simulink model "finalsimple_VER"  (R2023b)
settings: Solver=VariableStepAuto  StartTime=0.0  StopTime=5  FixedStep=4  MaxStep=0.01  RelTol=1e-3
undefined symbols (not defined in the file or in its folder): Ion, Lithium
libraries: simulink x40, nesl_utility x10, spsSeriesRLCBranchLib x8, fl_lib x6, spsMosfetLib x6, dspsrcs4 x5, spsControlledCurrentSourceLib x5, ee_lib x4, spsCurrentMeasurementLib x4, spsVoltageMeasurementLib x4, spsBatteryLib x3, spsGroundLib x2
(part 2 of 2)

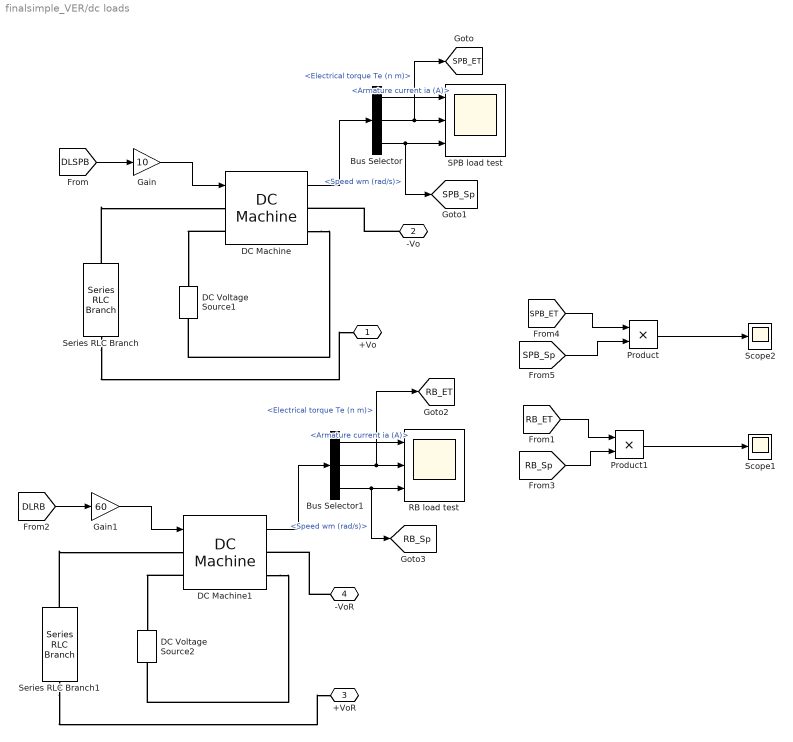
== system finalsimple_VER/dc loads ==
  Bus Selector : BusSelector  OutputSignals=Armature current ia (A),Electrical torque Te (n m),Speed wm (rad/s)
  Bus Selector1 : BusSelector  OutputSignals=Armature current ia (A),Electrical torque Te (n m),Speed wm (rad/s)
  DC Machine : spsDCMachineLib/DC Machine  PresetModel=No  MechanicalLoad=Speed w  FieldType=Wound  ShowDetailedParameters=on  MeasurementBus=off  RLa=[0.2828 0.004453]  RLf=[69.77 9.413]  Laf=0.5899  MachineConstant=Torque constant (N.m/A)  Ke=1.8  Kt=1.8  J=1.019  Bm=0.02516  Tf=26.46  w0=1  Ifinit=-8.59968467822847  TsPowergui=0  TsBlock=1
  DC Machine1 : spsDCMachineLib/DC Machine  PresetModel=No  MechanicalLoad=Speed w  FieldType=Wound  ShowDetailedParameters=on  MeasurementBus=off  RLa=[0.2828 0.004453]  RLf=[69.77 9.413]  Laf=0.5899  MachineConstant=Torque constant (N.m/A)  Ke=1.8  Kt=1.8  J=1.019  Bm=0.02516  Tf=26.46  w0=1  Ifinit=-4.29984233911423  TsPowergui=0  TsBlock=1
  DC Voltage Source1 : spsDCVoltageSourceLib/DC Voltage Source  Amplitude=600  Measurements=None
  DC Voltage Source2 : spsDCVoltageSourceLib/DC Voltage Source  Amplitude=300  Measurements=None
  Gain : Gain  Gain=10
  Gain1 : Gain  Gain=60
  Product : Product
  Product1 : Product
  RB load test : Scope  NumInputPorts=3
  SPB load test : Scope  NumInputPorts=3
  Scope1 : Scope
  Scope2 : Scope
  Series RLC Branch : spsSeriesRLCBranchLib/Series RLC Branch  LConnTagsString=__new0  RConnTagsString=__new0  BranchType=R  Resistance=1e3  Inductance=1e-3  SetiL0=off  InitialCurrent=0  Capacitance=1e-6  Setx0=off  InitialVoltage=0  Measurements=None
  Series RLC Branch1 : spsSeriesRLCBranchLib/Series RLC Branch  LConnTagsString=__new0  RConnTagsString=__new0  BranchType=R  Resistance=1e3  Inductance=1e-3  SetiL0=off  InitialCurrent=0  Capacitance=1e-6  Setx0=off  InitialVoltage=0  Measurements=None
  +Vo : PMIOPort  Side=Right
  -Vo : PMIOPort  Port=2  Side=Right
  +VoR : PMIOPort  Port=3  Side=Right
  -VoR : PMIOPort  Port=4  Side=Right
  tag scope: RB_ET=global, RB_Sp=global, SPB_ET=global, SPB_Sp=global
  wires:
  Bus Selector/3 -> SPB load test/3, [SPB_Sp]  "<Speed wm (rad/s)>"
  Bus Selector/2 -> [SPB_ET], SPB load test/2  "<Electrical torque Te (n m)>"
  DC Machine/1 -> Bus Selector/1
  Bus Selector/1 -> SPB load test/1  "<Armature current ia (A)>"
  [DLSPB] -> Gain/1
  [DLRB] -> Gain1/1
  Bus Selector1/1 -> RB load test/1  "<Armature current ia (A)>"
  DC Machine1/1 -> Bus Selector1/1
  Bus Selector1/2 -> [RB_ET], RB load test/2  "<Electrical torque Te (n m)>"
  Bus Selector1/3 -> [RB_Sp], RB load test/3  "<Speed wm (rad/s)>"
  Gain1/1 -> DC Machine1/1
  Gain/1 -> DC Machine/1
  [SPB_ET] -> Product/1
  [SPB_Sp] -> Product/2
  Product/1 -> Scope2/1
  Product1/1 -> Scope1/1
  [RB_ET] -> Product1/1
  [RB_Sp] -> Product1/2
  connections:
  -Vo/RConn1 -- DC Machine/RConn1
  DC Machine/RConn2 -- DC Voltage Source1/RConn1
  DC Machine/LConn2 -- DC Voltage Source1/LConn1
  Series RLC Branch/LConn1 -- DC Machine/LConn1
  Series RLC Branch1/LConn1 -- DC Machine1/LConn1
  DC Machine1/LConn2 -- DC Voltage Source2/LConn1
  DC Machine1/RConn2 -- DC Voltage Source2/RConn1
  -VoR/RConn1 -- DC Machine1/RConn1
  Series RLC Branch/RConn1 -- +Vo/RConn1
  Series RLC Branch1/RConn1 -- +VoR/RConn1

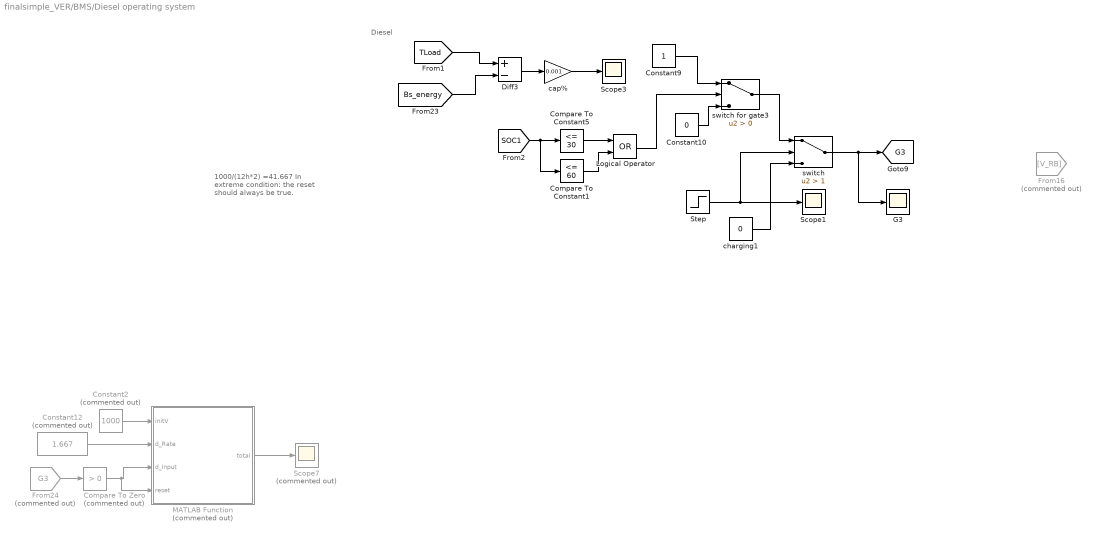
== system finalsimple_VER/BMS/Diesel operating system ==
  note: Diesel
  note: 1000/(12h*2)
      | =41.667
      |
      | In extreme condition:
      | the reset should
      | always be true.
  Compare To Constant1 : simulink/Logic and Bit Operations/Compare To Constant  relop=<=  const=60  OutDataTypeStr=boolean
  Compare To Constant5 : simulink/Logic and Bit Operations/Compare To Constant  relop=<=  const=30  OutDataTypeStr=boolean
  Compare To Zero : simulink/Logic and Bit Operations/Compare To Zero  Commented=on  relop=>  OutDataTypeStr=boolean
  Constant10 : Constant  Value=0
  Constant12 : Constant  Commented=on  Value=1.667
  Constant2 : Constant  Commented=on  Value=1000
  Constant9 : Constant
  Diff3 : Sum  Inputs=+-
  From16 : From  Commented=on  GotoTag=V_RB  TagVisibility=global
  From24 : From  Commented=on  GotoTag=G3  TagVisibility=global
  G3 : Scope
  Logical Operator : Logic  Operator=OR  AllPortsSameDT=off  OutDataTypeStr=boolean
  MATLAB Function : MATLAB Function  Commented=on  TreatAsAtomicUnit=on
  Scope1 : Scope
  Scope3 : Scope
  Scope7 : Scope  Commented=on
  Step : Step  Time=2400  After=2  SampleTime=1
  cap% : Gain  Gain=0.001
  charging1 : Constant  Value=0
  "switch " : Switch  Criteria=u2 > Threshold  Threshold=1  SaturateOnIntegerOverflow=off  InputSameDT=off
  switch for gate3 : Switch  Criteria=u2 > Threshold  SaturateOnIntegerOverflow=off  InputSameDT=off
  tag scope: G3=global
  wires:
  Constant9/1 -> switch for gate3/1
  Constant10/1 -> switch for gate3/3
  Constant12/1 -> MATLAB Function/2(d_Rate)
  MATLAB Function/1(total) -> Scope7/1
  Compare To Zero/1 -> MATLAB Function/4(reset), MATLAB Function/3(d_Input)
  From24/1 -> Compare To Zero/1
  Diff3/1 -> cap%/1
  Constant2/1 -> MATLAB Function/1(initV)
  [TLoad] -> Diff3/1
  Step/1 -> "switch "/2, Scope1/1
  charging1/1 -> "switch "/3
  "switch "/1 -> [G3], G3/1
  switch for gate3/1 -> "switch "/1
  [Bs_energy] -> Diff3/2
  [SOC1] -> Compare To Constant1/1, Compare To Constant5/1
  cap%/1 -> Scope3/1
  Compare To Constant1/1 -> Logical Operator/2
  Compare To Constant5/1 -> Logical Operator/1
  Logical Operator/1 -> switch for gate3/2

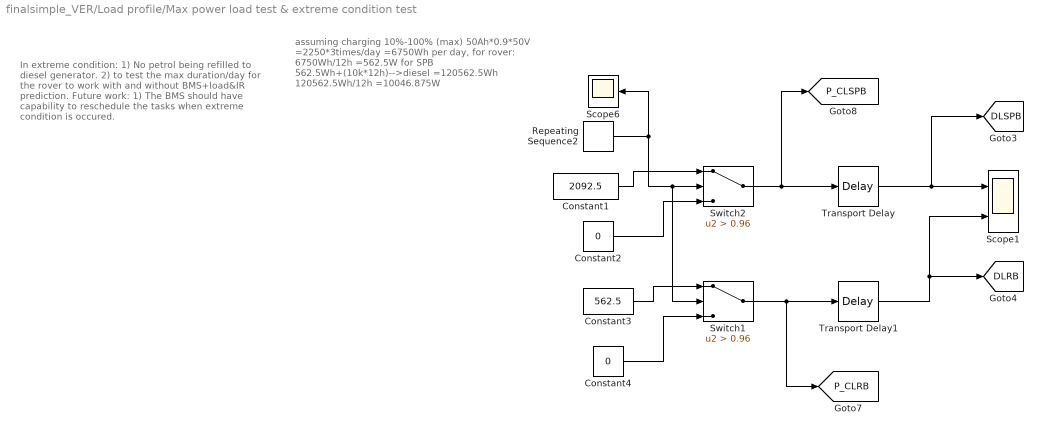
== system finalsimple_VER/Load profile/Max power load test & extreme condition test ==
  note: assuming charging 10%-100% (max)
      | 50Ah*0.9*50V
      | =2250*3times/day
      | =6750Wh per day,
      | for rover:
      | 6750Wh/12h
      | =562.5W
      |
      | for SPB
      | 562.5Wh+(10k*12h)-->diesel
      | =120562.5Wh
      |
      | 120562.5Wh/12h
      | =10046.875W
  note: In extreme condition:
      | 1) No petrol being refilled
      | to diesel generator.
      | 2) to test the max duration/day for
      | the rover to work with
      | and without BMS+load&IR prediction.
      |
      | Future work:
      | 1) The BMS should have capability
      | to reschedule the tasks when
      | extreme condition is occured.
  Constant1 : Constant  Value=2092.5
  Constant2 : Constant  Value=0
  Constant3 : Constant  Value=562.5
  Constant4 : Constant  Value=0
  Repeating Sequence2 : simulink/Sources/Repeating Sequence  rep_seq_t=[0 300 300.1 900.99 901 1200]  rep_seq_y=[0.9 0.9 1.01 1.01 0.9 0.9]
  Scope1 : Scope  NumInputPorts=2
  Scope6 : Scope
  Switch1 : Switch  Criteria=u2 > Threshold  Threshold=0.96  RndMeth=Ceiling  ZeroCross=off  SaturateOnIntegerOverflow=off
  Switch2 : Switch  Criteria=u2 > Threshold  Threshold=0.96  RndMeth=Ceiling  ZeroCross=off  SaturateOnIntegerOverflow=off
  Transport Delay : TransportDelay  DelayTime=2400
  Transport Delay1 : TransportDelay  DelayTime=2400
  tag scope: DLRB=global, DLSPB=global, P_CLRB=global, P_CLSPB=global
  wires:
  Switch1/1 -> [P_CLRB], Transport Delay1/1
  Switch2/1 -> [P_CLSPB], Transport Delay/1
  Repeating Sequence2/1 -> Scope6/1, Switch1/2, Switch2/2
  Constant2/1 -> Switch2/3
  Constant1/1 -> Switch2/1
  Constant3/1 -> Switch1/1
  Constant4/1 -> Switch1/3
  Transport Delay/1 -> [DLSPB], Scope1/1
  Transport Delay1/1 -> Scope1/2, [DLRB]

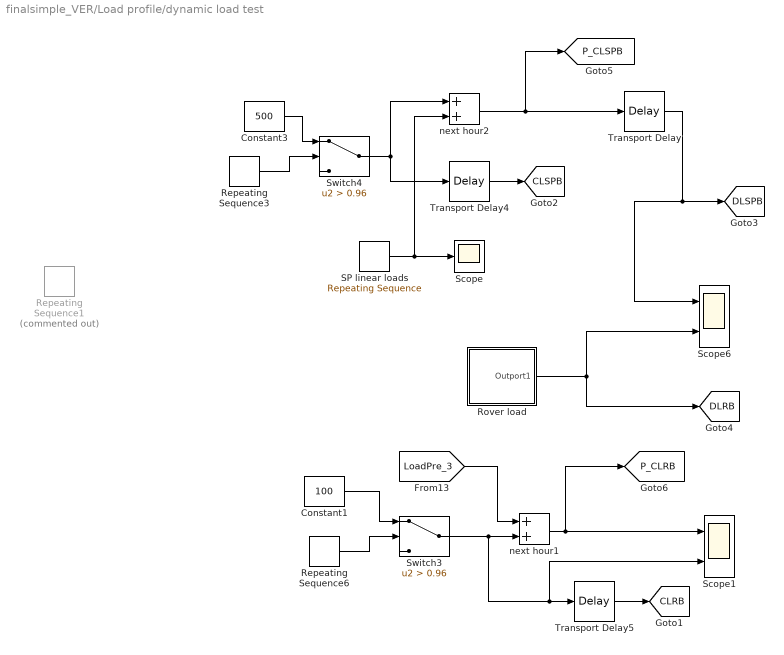
== system finalsimple_VER/Load profile/dynamic load test ==
  Constant1 : Constant  Value=100
  Constant3 : Constant  Value=500
  Repeating Sequence1 : simulink/Sources/Repeating Sequence  Commented=on  rep_seq_t=[0 400 500 600 700 800 900 1000 1200]  rep_seq_y=[0 0 1000 800 1000 800 500 0 0]
  Repeating Sequence3 : simulink/Sources/Repeating Sequence  rep_seq_t=[0 300 300.1 900.99 901 1200]  rep_seq_y=[0.9 0.9 1.01 1.01 0.9 0.9]
  Repeating Sequence6 : simulink/Sources/Repeating Sequence  rep_seq_t=[0 300 300.1 900.99 901 1200]  rep_seq_y=[0.9 0.9 1.01 1.01 0.9 0.9]
  Rover load : Subsystem
  SP linear loads : simulink/Sources/Repeating Sequence  rep_seq_t=[0 400 401 500 501 600 601 700 701 800 900 1000 1001 1200]  rep_seq_y=[0 0 1000 1000 800 800 1000 1000 800 800 500 500 0 0]
  Scope : Scope
  Scope1 : Scope  NumInputPorts=2
  Scope6 : Scope  NumInputPorts=2
  Switch3 : Switch  Criteria=u2 > Threshold  Threshold=0.96  RndMeth=Ceiling  ZeroCross=off  SaturateOnIntegerOverflow=off
  Switch4 : Switch  Criteria=u2 > Threshold  Threshold=0.96  RndMeth=Ceiling  ZeroCross=off  SaturateOnIntegerOverflow=off
  Transport Delay : TransportDelay  DelayTime=2400
  Transport Delay4 : TransportDelay  DelayTime=2400
  Transport Delay5 : TransportDelay  DelayTime=2400
  next hour1 : Sum
  next hour2 : Sum
  tag scope: CLRB=global, CLSPB=global, DLRB=global, DLSPB=global, P_CLRB=global, P_CLSPB=global
  wires:
  SP linear loads/1 -> next hour2/2, Scope/1
  Rover load/1(Outport1) -> Scope6/2, [DLRB]
  Transport Delay/1 -> Scope6/1, [DLSPB]
  Repeating Sequence6/1 -> Switch3/2
  Constant3/1 -> Switch4/1
  Constant1/1 -> Switch3/1
  Transport Delay5/1 -> [CLRB]
  Transport Delay4/1 -> [CLSPB]
  Repeating Sequence3/1 -> Switch4/2
  Switch4/1 -> Transport Delay4/1, next hour2/1
  [LoadPre_3] -> next hour1/1
  next hour1/1 -> [P_CLRB], Scope1/1
  next hour2/1 -> [P_CLSPB], Transport Delay/1
  Switch3/1 -> Scope1/2, Transport Delay5/1, next hour1/2

== system finalsimple_VER/Load profile/small load test ==
  Constant1 : Constant
  Constant3 : Constant
  tag scope: DLRB=global, DLSPB=global
  wires:
  Constant1/1 -> [DLSPB]
  Constant3/1 -> [DLRB]

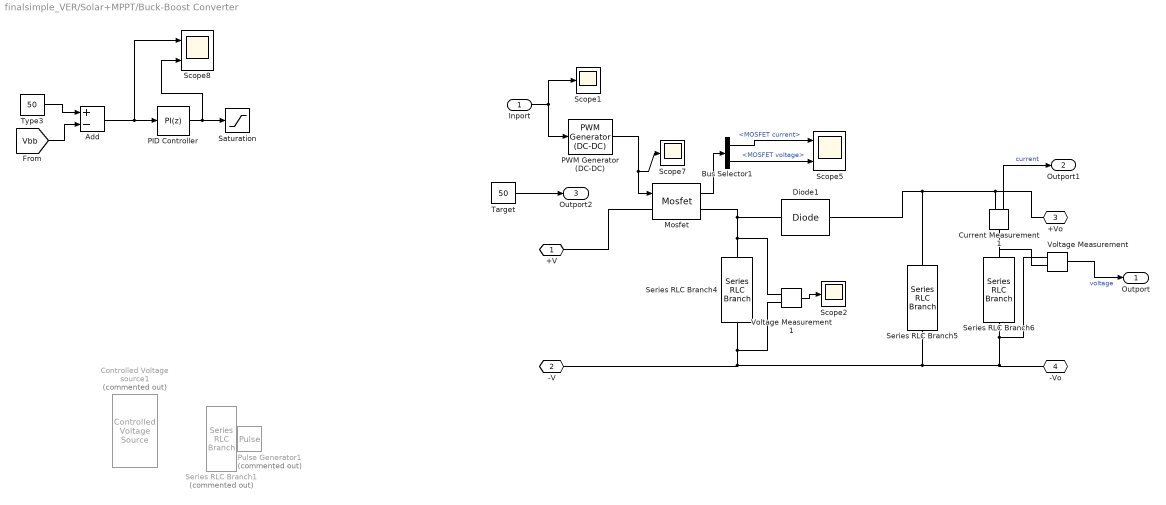
== system finalsimple_VER/Solar+MPPT/Buck-Boost Converter ==
  Inport : Inport
  Add : Sum  Inputs=+-
  Bus Selector1 : BusSelector  OutputSignals=MOSFET current,MOSFET voltage
  Controlled Voltage source1 : spsControlledVoltageSourceLib/Controlled Voltage Source  Commented=on  Initialize=on  Source_Type=DC  Amplitude=0  Phase=0  Frequency=0  Measurements=None
  Current Measurement1 : spsCurrentMeasurementLib/Current Measurement  PhasorSimulation=off  OutputType=Complex  PSBequivalent=0
  Diode1 : spsDiodeLib/Diode  Ron=0.001  Lon=0  Vf=0.8  IC=0  UseSnubber=0  Rs=500  Cs=250e-9  Measurements=off
  Mosfet : spsMosfetLib/Mosfet  Ron=0.1  Lon=0  Rd=0.01  Vfd=0  IC=0  Rs=1e5  Cs=inf  Measurements=on
  PID Controller : slpidlib/PID Controller  Controller=PI  Form=Parallel  TimeDomain=Discrete-time  UseExternalTs=off  SampleTime=-1  IntegratorMethod=Forward Euler  FilterMethod=Forward Euler  ControllerParametersSource=internal  P=0.448206848938492  I=8.01083955194228  UseKiTs=off  D=0  N=100  UseFilter=on  TunerSelectOption=Transfer Function Based (PID Tuner App)  InitialConditionSource=internal  InitialConditionForIntegrator=0  InitialConditionForFilter=0  DifferentiatorICPrevScaledInput=0  ExternalReset=none  TrackingMode=off  Kt=1  LimitOutput=on  SatLimitsSource=internal  UpperSaturationLimit=0.8  LowerSaturationLimit=0  LinearizeAsGain=off  AntiWindupMode=none  Kb=1  LimitIntegrator=on  UpperIntegratorSaturationLimit=0.8  LowerIntegratorSaturationLimit=0  POutMin=[]  POutMax=[]  IOutMin=[]  IOutMax=[]  DOutMin=[]  DOutMax=[]  NOutMin=[]  NOutMax=[]  SumOutMin=[]  SumOutMax=[]  SaturationOutMin=[]  SaturationOutMax=[]  PParamMin=[]  PParamMax=[]  IParamMin=[]  IParamMax=[]  DParamMin=[]  DParamMax=[]  NParamMin=[]  NParamMax=[]  KbParamMin=[]  KbParamMax=[]  KtParamMin=[]  KtParamMax=[]  KbOutMin=[]  KbOutMax=[]  KtOutMin=[]  KtOutMax=[]  IntegratorOutMin=[]  IntegratorOutMax=[]  FilterOutMin=[]  FilterOutMax=[]  SumI1OutMin=[]  SumI1OutMax=[]  SumI2OutMin=[]  SumI2OutMax=[]  SumI3OutMin=[]  SumI3OutMax=[]  SumI4OutMin=[]  SumI4OutMax=[]  SumDOutMin=[]  SumDOutMax=[]  DifferentiatorOutMin=[]  DifferentiatorOutMax=[]  FilterDiffOutCoefMin=[]  FilterDiffOutCoefMax=[]  ReciprocalOutMin=[]  ReciprocalOutMax=[]  SumDenOutMin=[]  SumDenOutMax=[]  SumNumOutMin=[]  SumNumOutMax=[]  DivideOutMin=[]  DivideOutMax=[]  UdiffTsProdOutMin=[]  UdiffTsProdOutMax=[]  NTsProdOutMin=[]  NTsProdOutMax=[]  UintegralTsProdOutMin=[]  UintegralTsProdOutMax=[]  UngainTsProdOutMin=[]  UngainTsProdOutMax=[]  ClampingZeroOutDataTypeStr=Inherit: Inherit via back propagation  ClampingZeroOutMin=[]  ClampingZeroOutMax=[]  FilterDenConstantOutDataTypeStr=Inherit: Inherit via back propagation  FilterDenConstantOutMin=[]  FilterDenConstantOutMax=[]  PCopyOutDataTypeStr=Inherit: Inherit via back propagation  PCopyOutMin=[]  PCopyOutMax=[]  NCopyOutDataTypeStr=Inherit: Inherit via back propagation  NCopyOutMin=[]  NCopyOutMax=[]  IntegratorContinuousStateAttributes=''  IntegratorStateMustResolveToSignalObject=off  IntegratorRTWStateStorageClass=Auto  FilterContinuousStateAttributes=''  FilterStateMustResolveToSignalObject=off  FilterRTWStateStorageClass=Auto  ParallelPVariant=InternalParameters  IdealPVariant=Disabled  IVariant=InternalParameters  DVariant=Disabled  IntegratorVariant=Discrete  SatVariant=Enabled  AWVariant=Passthrough  PCopyVariant=Disabled  TRVariant=Disabled  FdbkBlocksVariant=Forward  IdealPFdbkVariant=Disabled  SatFdbkVariant=Disabled  DerivativeFilterVariant=Disabled  NVariant=Disabled  NCopyVariant=Disabled_SignalSpec  FilterICVariant=Disabled  IntegratorICVariant=InternalICs  ExternalResetVariant=Disabled  TRSumVariant=Passthrough  SumFdbkVariant=Disabled  SumVariant=Sum_PI  TsampFilterVariant=InternalTs  TsampNgainVariant=Passthrough  TsampIntegralVariant=Disabled_SignalSpec  ExternalSaturationOutDataTypeStr=Inherit: Same as second input
  PWM Generator (DC-DC) : spsPWMGeneratorDCDCLib/PWM Generator (DC-DC)  Fsw=3500  Ts=0
  Pulse Generator1 : DiscretePulseGenerator  Commented=on  Period=10  PulseWidth=8  SampleTime=5e-6
  Saturation : Saturate  UpperLimit=0.8  LowerLimit=0
  Scope1 : Scope
  Scope2 : Scope
  Scope5 : Scope  NumInputPorts=2
  Scope7 : Scope
  Scope8 : Scope  NumInputPorts=2
  Series RLC Branch1 : spsSeriesRLCBranchLib/Series RLC Branch  Commented=on  LConnTagsString=__new0  RConnTagsString=__new0  BranchType=L  Resistance=1  Inductance=8e-2  SetiL0=off  InitialCurrent=0  Capacitance=1e-6  Setx0=off  InitialVoltage=0  Measurements=None
  Series RLC Branch4 : spsSeriesRLCBranchLib/Series RLC Branch  LConnTagsString=__new0  RConnTagsString=__new0  BranchType=L  Resistance=1  Inductance=1e-3  SetiL0=off  InitialCurrent=0  Capacitance=1e-6  Setx0=off  InitialVoltage=0  Measurements=None
  Series RLC Branch5 : spsSeriesRLCBranchLib/Series RLC Branch  LConnTagsString=__new0  RConnTagsString=__new0  BranchType=C  Resistance=1  Inductance=1e-3  SetiL0=off  InitialCurrent=0  Capacitance=1e-1  Setx0=off  InitialVoltage=0  Measurements=None
  Series RLC Branch6 : spsSeriesRLCBranchLib/Series RLC Branch  LConnTagsString=__new0  RConnTagsString=__new0  BranchType=R  Resistance=10  Inductance=1e-3  SetiL0=off  InitialCurrent=0  Capacitance=1e-6  Setx0=off  InitialVoltage=0  Measurements=None
  Target : Constant  Value=50  SampleTime=0
  Type3 : Constant  Value=50  SampleTime=0
  Voltage Measurement : spsVoltageMeasurementLib/Voltage Measurement  PhasorSimulation=off  OutputType=Complex  PSBequivalent=0
  Voltage Measurement1 : spsVoltageMeasurementLib/Voltage Measurement  PhasorSimulation=off  OutputType=Complex  PSBequivalent=0
  +V : PMIOPort  Side=Left
  -V : PMIOPort  Port=2  Side=Left
  +Vo : PMIOPort  Port=3  Side=Right
  -Vo : PMIOPort  Port=4  Side=Right
  Outport : Outport
  Outport1 : Outport  Port=2
  Outport2 : Outport  Port=3
  wires:
  [Vbb] -> Add/2
  Voltage Measurement/1 -> Outport/1  "voltage"
  Bus Selector1/1 -> Scope5/1  "<MOSFET current>"
  Voltage Measurement1/1 -> Scope2/1
  Bus Selector1/2 -> Scope5/2  "<MOSFET voltage>"
  PID Controller/1 -> Scope8/2, Saturation/1
  Add/1 -> Scope8/1, PID Controller/1
  Type3/1 -> Add/1
  PWM Generator (DC-DC)/1 -> Mosfet/1, Scope7/1
  Mosfet/1 -> Bus Selector1/1
  Inport/1 -> Scope1/1, PWM Generator (DC-DC)/1
  Current Measurement1/1 -> Outport1/1  "current"
  Target/1 -> Outport2/1
  connections:
  Mosfet/RConn1 -- Diode1/RConn1 -- Voltage Measurement1/LConn1 -- Series RLC Branch4/LConn1
  Series RLC Branch6/LConn1 -- Voltage Measurement/LConn2 -- Current Measurement1/LConn1
  +V/RConn1 -- Mosfet/LConn1
  Series RLC Branch5/LConn1 -- Diode1/LConn1 -- +Vo/RConn1 -- Current Measurement1/RConn1
  Series RLC Branch6/RConn1 -- Voltage Measurement/LConn1 -- Series RLC Branch5/RConn1 -- Series RLC Branch4/RConn1 -- Voltage Measurement1/LConn2 -- -V/RConn1 -- -Vo/RConn1

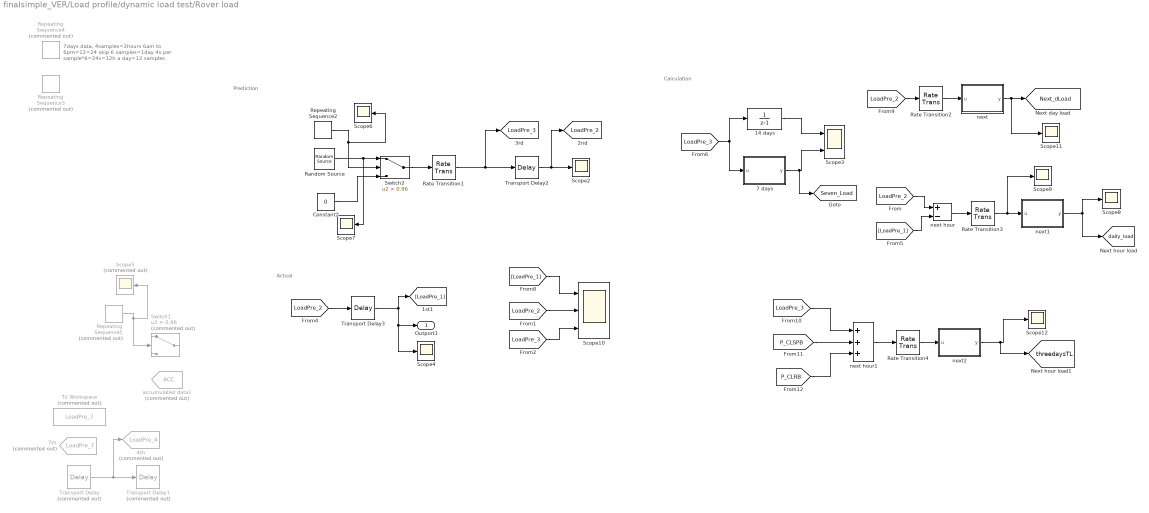
== system finalsimple_VER/Load profile/dynamic load test/Rover load ==
  note: 7days data,
      | 4samples=2hours
      | 6am to 6pm=12=24
      | skip 6 samples=1day
      | 4s per sample*6=24s=12h
      | a day=12 samples
  note: Calculation
  note: Prediction
  note: Actual
  14 days : DiscreteTransferFcn  Denominator=[1 -1]  a0EqualsOne=on
  4th : Goto  Commented=on  GotoTag=LoadPre_4  TagVisibility=global
  7 days : MATLAB Function  TreatAsAtomicUnit=on
  7th : Goto  Commented=on  GotoTag=LoadPre_7  TagVisibility=global
  Constant2 : Constant  Value=0
  Random Source : dspsrcs4/Random Source  SrcType=Uniform  NormMethod=Ziggurat  CltLength=12  MinVal=0  MaxVal=500  MeanVal=0  VarVal=1  RepMode=Not repeatable  rawSeed=1  IsInherit=off  SampMode=Discrete  SampTime=50  SampFrame=1  DataType=Double  OutComplex=Real  OutputFrames=off
  Rate Transition1 : RateTransition  OutPortSampleTime=100
  Rate Transition2 : RateTransition  OutPortSampleTime=50
  Rate Transition3 : RateTransition  OutPortSampleTime=100
  Rate Transition4 : RateTransition  OutPortSampleTime=100
  Repeating Sequence2 : simulink/Sources/Repeating Sequence  rep_seq_t=[0 250 250.1 899.99 900 1200]  rep_seq_y=[0.9 0.9 1.01 1.01 0.9 0.9]
  Repeating Sequence3 : simulink/Sources/Repeating Sequence  Commented=on  rep_seq_t=[0 12 12.1 71.99 72 96]  rep_seq_y=[0.9 0.9 1.01 1.01 0.9 0.9]
  Repeating Sequence4 : simulink/Sources/Repeating Sequence  Commented=on  rep_seq_t=[0 16 16.1 71.99 72 96]  rep_seq_y=[0.9 0.9 1.01 1.01 0.9 0.9]
  Repeating Sequence5 : simulink/Sources/Repeating Sequence  Commented=on  rep_seq_t=[0 300 300.1 900.99 901 1200]  rep_seq_y=[0.9 0.9 1.01 1.01 0.9 0.9]
  Scope10 : Scope  NumInputPorts=3
  Scope{2,4,6..9,11..12} (8 alike) : Scope
  Scope3 : Scope  NumInputPorts=2
  Scope5 : Scope  Commented=on
  Switch1 : Switch  Commented=on  Criteria=u2 > Threshold  Threshold=0.96  RndMeth=Ceiling  ZeroCross=off  SaturateOnIntegerOverflow=off
  Switch2 : Switch  Criteria=u2 > Threshold  Threshold=0.96  RndMeth=Ceiling  ZeroCross=off  SaturateOnIntegerOverflow=off
  To Workspace : ToWorkspace  Commented=on  VariableName=LoadPre_7  SaveFormat=Structure With Time  SampleTime=1
      settings: Decimation=2  Save2DSignal=2-D array (concatenate along first dimension)
  Transport Delay : TransportDelay  Commented=on  DelayTime=288
  Transport Delay1 : TransportDelay  Commented=on  DelayTime=96
  Transport Delay2 : TransportDelay  DelayTime=1200
  Transport Delay3 : TransportDelay  DelayTime=1200
  accumulated data1 : Goto  Commented=on  GotoTag=ACC  TagVisibility=global
  next : MATLAB Function  TreatAsAtomicUnit=on
  next hour : Sum  Inputs=+-
  next hour1 : Sum  Inputs=+++
  next1 : MATLAB Function  TreatAsAtomicUnit=on
  next2 : MATLAB Function  TreatAsAtomicUnit=on
  Outport1 : Outport
  tag scope: LoadPre_2=global, LoadPre_3=global, Next_dLoad=global, Seven_Load=global, daily_load=global, threedaysTL=global
  wires:
  Transport Delay2/1 -> Scope2/1, [LoadPre_2]
  Switch2/1 -> Rate Transition1/1
  [LoadPre_3] -> Scope10/3
  [LoadPre_2] -> Rate Transition2/1
  Repeating Sequence2/1 -> Scope6/1, Switch2/2
  Constant2/1 -> Switch2/3
  [LoadPre_2] -> Transport Delay3/1
  [LoadPre_2] -> next hour/1
  [LoadPre_3] -> 7 days/1(u), 14 days/1
  Random Source/1 -> Switch2/1, Scope7/1
  14 days/1 -> Scope3/1
  [LoadPre_1] -> next hour/2
  Transport Delay/1 -> 4th/1, Transport Delay1/1
  7 days/1(y) -> [Seven_Load], Scope3/2
  [LoadPre_1] -> Scope10/1
  [LoadPre_2] -> Scope10/2
  Transport Delay3/1 -> Scope4/1, Outport1/1, [LoadPre_1]
  Repeating Sequence5/1 -> Switch1/2, Scope5/1
  ? -> accumulated data1/1, Switch1/1
  ? -> Switch1/3
  next/1(y) -> Scope11/1, [Next_dLoad]
  Rate Transition2/1 -> next/1(u)
  Rate Transition3/1 -> Scope9/1, next1/1(u)
  next hour/1 -> Rate Transition3/1
  next1/1(y) -> [daily_load], Scope8/1
  [LoadPre_3] -> next hour1/1
  [P_CLSPB] -> next hour1/2
  [P_CLRB] -> next hour1/3
  next hour1/1 -> Rate Transition4/1
  Rate Transition4/1 -> next2/1(u)
  next2/1(y) -> [threedaysTL], Scope12/1
  Rate Transition1/1 -> [LoadPre_3], Transport Delay2/1

== matlab function finalsimple_VER/BMS/total PIR ==
  data: u input; y output
function y = fcn(u)
    
    persistent a sampleCount
    if isempty(a)
        a = 0;
        sampleCount = 0;
    end
    
    % Update the output and the accumulated value
    y = u + a;
    a = y;
    
    % Increment the sample counter
    sampleCount = sampleCount + 1;
    
    % Reset the accumulation after 
    %24 samples per day.
    if sampleCount >= 12 
        a = 0;
        sampleCount = 0;
    end
end

== matlab function finalsimple_VER/BMS/Diesel operating system/MATLAB Function ==
  data: initV input; total output; d_Rate input; d_Input input; reset input
function total = Diesel_CAP(initV, d_Rate, d_Input, reset)
    
%R=remaining
    persistent R timeStep
    
    if isempty(R)
        R = initV;
        timeStep = 0;
    end
    
    
    if reset==false
        R = initV;
        timeStep = 0;
    elseif d_Input
        % Decrease the total value linearly 
        R = initV - d_Rate * timeStep;
        timeStep = timeStep + 1;
        
        % Ensure the value does not go below 0
        if R < 0
            R = 0;
        end
    end
    % Output the value
    total = R;
end

== matlab function finalsimple_VER/Load profile/dynamic load test/Rover load/next1 ==
  data: u input; y output
function y = fcn(u)
    
    persistent a sampleCount
    if isempty(a)
        a = 0;
        sampleCount = 0;
    end
    
    % Update the output and the accumulated value
    y = u + a;
    a = y;
    
    % Increment the sample counter
    sampleCount = sampleCount + 1;
    
    % Reset the accumulation after 24 samples
    if sampleCount >= 12
        a = 0;
        sampleCount = 0;
    end
end

== matlab function finalsimple_VER/Load profile/dynamic load test/Rover load/next2 ==
  data: u input; y output
function y = fcn(u)
    
    persistent a sampleCount
    if isempty(a)
        a = 0;
        sampleCount = 0;
    end
    
    % Update the output and the accumulated value
    y = u + a;
    a = y;
    
    % Increment the sample counter
    sampleCount = sampleCount + 1;
    
    % Reset the accumulation after 24 samples
    if sampleCount >= 12
        a = 0;
        sampleCount = 0;
    end
end

== matlab function finalsimple_VER/BMS/total SOC1 ==
  data: u input; y output
function y = fcn(u)
    
    persistent a sampleCount
    if isempty(a)
        a = 0;
        sampleCount = 0;
    end
    
    % Update the output and the accumulated value
    y = u + a;
    a = y;
    
    % Increment the sample counter
    sampleCount = sampleCount + 1;
    
    % Reset the accumulation after 
    %24 samples per day.
    if sampleCount >= 84
        a = 0;
        sampleCount = 0;
    end
end

== matlab function finalsimple_VER/BMS/total SOC2 ==
  data: u input; y output
function y = fcn(u)
    
    persistent a sampleCount
    if isempty(a)
        a = 0;
        sampleCount = 0;
    end
    
    % Update the output and the accumulated value
    y = u + a;
    a = y;
    
    % Increment the sample counter
    sampleCount = sampleCount + 1;
    
    % Reset the accumulation after 
    %24 samples per day.
    if sampleCount >= 84
        a = 0;
        sampleCount = 0;
    end
end

== matlab function finalsimple_VER/BMS/total charge rate ==
  data: u input; y output
function y = fcn(u)
    
    persistent a sampleCount
    if isempty(a)
        a = 0;
        sampleCount = 0;
    end
    
    % Update the output and the accumulated value
    y = u + a;
    a = y;
    
    % Increment the sample counter
    sampleCount = sampleCount + 1;
    
    % Reset the accumulation after 
    %24 samples per day.
    if sampleCount >= 12
        a = 0;
        sampleCount = 0;
    end
end

== matlab function finalsimple_VER/BMS/total SOC ==
  data: u input; y output
function y = fcn(u)
    
    persistent a sampleCount
    if isempty(a)
        a = 0;
        sampleCount = 0;
    end
    
    % Update the output and the accumulated value
    y = u + a;
    a = y;
    
    % Increment the sample counter
    sampleCount = sampleCount + 1;
    
    % Reset the accumulation after 
    %24 samples per day.
    if sampleCount >= 84
        a = 0;
        sampleCount = 0;
    end
end

== matlab function finalsimple_VER/BMS/total PIR1 ==
  data: u input; y output
function y = fcn(u)
    
    persistent a sampleCount
    if isempty(a)
        a = 0;
        sampleCount = 0;
    end
    
    % Update the output and the accumulated value
    y = u + a;
    a = y;
    
    % Increment the sample counter
    sampleCount = sampleCount + 1;
    
    % Reset the accumulation after 
    %24 samples per day.
    if sampleCount >= 12 
        a = 0;
        sampleCount = 0;
    end
end

== matlab function finalsimple_VER/Solar+MPPT/Algorithm1 ==
  settings: updateMethod=DISCRETE
  data: Type input; I input; Vmpp output; V input; Pmpp output; deltaV output; gpast input; gnext output; duty output; target input; Vbb input; check_old output; deltaw output
function [Vmpp,Pmpp,deltaV, gnext, duty, check_old,deltaw] = MPPT(Type,I,V,gpast, target, Vbb)

duty_init = 0.3;
check=0;
% min and max value are used to limit duty between
% 0 and 0.85
delta=1e-4; %in steady state
duty_min=0;
duty_max=0.85;
duty=0.3;


persistent Vpast Ipast Ppast duty_old;
    if isempty(Vpast) % Setup some initial values
        Vpast=0.000001;
        Ipast=0.000001;
        
        %gpast=1;
        duty_old=duty_init;
        Ppast=Vpast*Ipast;
    end

deltaV=0; % initializing
P= V*I; % Measure Power for current iteration 
dI= I - Ipast;
dV= V - Vpast;
dP= P - Ppast;
g=abs(dP);
gpast=abs(gpast);
gup=gpast*1.2;
glow=gpast*0.8;

%% Define DeltaV for fixed perturbation-step MPPT [1]
    if (Type==1)  
        % suggested range of M;  0.3 @ 1000m/m2 and 0.7 @ 200m/m2
        delta = delta;

    %%%%%%%%%%%%%%%%%%%%%%%%%%%%%%%%%%%%%%%%%%%%%%%%%%%%%%%%%%
    elseif (Type ==2)
        if (g>=glow && g<gup)
            delta=delta;   %used to track linear mpp
            check=-1;
        elseif g>= gup
            %deltaV=3.41*abs(dI*V*(dV/dP));
            delta=(1e-4)*abs(dV*I*(dI/dP));  %used to track curve mpp          
            check=1;
        else
            delta=0;
        end
    end

%% MPPT Algorithm  
if dP ~= 0
    if dP < 0
        if dV < 0
            Vmpp = V + deltaV;
            if Vbb < target
                duty=duty_old + delta;
            elseif Vbb > target
                duty=duty_old - delta;
            else
                duty=duty_old;
            end
        else
            Vmpp = V - deltaV;
            if Vbb < target
                duty=duty_old + delta;
            elseif Vbb > target
                duty=duty_old - delta;
            else
                duty=duty_old;
            end
        end
    else
        if dV < 0
            Vmpp = V - deltaV;
            if Vbb < target
                duty=duty_old + delta;
            elseif Vbb > target
                duty=duty_old - delta;
            else
                duty=duty_old;
            end
        else
            Vmpp = V + deltaV;
            if Vbb < target
                duty=duty_old + delta;
            elseif Vbb > target
                duty=duty_old - delta;
            else
                duty=duty_old;
            end
        end    
    end
else
    Vmpp = V;
    duty=duty_old;
end


%the below if limits the duty between min and max
if duty > duty_max
    duty=duty_max;
elseif duty<duty_min
    duty=duty_min;
end     

Pmpp=Vmpp*I;

%%
% Update Past values
duty_old=duty;
Vpast=V;
Ppast=P;
Ipast=I;
gnext = g;
check_old=check;
deltaw=delta;
end

== matlab function finalsimple_VER/BMS/irradiance per day ==
  data: u input; y output
function y = fcn(u)
    
    persistent a sampleCount
    if isempty(a)
        a = 0;
        sampleCount = 0;
    end
      
    y = u + a;
    a = y;
    
    sampleCount = sampleCount + 1;
    
    % Reset
    if sampleCount >= 12 
        a = 0;
        sampleCount = 0;
    end
end

== matlab function finalsimple_VER/Solar+MPPT/Algorithm ==
  settings: updateMethod=DISCRETE
  data: Type input; I input; V input; duty output; target input; Vbb input; deltaw output
function [duty, deltaw] = MPPT(Type, I, V,target, Vbb)

    duty_init = 0.3;
    delta = 1e-3; % steady state step size
    duty_min = 0;
    duty_max = 0.85;
    duty = duty_init;
    deltaw=0;

    persistent Vpast Ipast Ppast duty_old;
    if isempty(Vpast) % Initialize persistent variables
        Vpast = 1e-6;
        Ipast = 1e-6;
        duty_old = duty_init;
        Ppast = Vpast * Ipast;
    end

    % Calculate current power and changes in current and voltage
    P = V * I;
    dI = I - Ipast;
    dV = V - Vpast;
    dP = P - Ppast;


    if Type==1  
        % suggested range of M;  0.3 @ 1000m/m2 and 0.7 @ 200m/m2
        delta = delta;

    elseif Type == 2
        
        if dP==0
            delta=0;
        else
            delta=(1e-3)*(dI/dP); % track curve MPP
            check = 1;
        end

    end

    % Determine new Vmpp and adjust duty cycle
    if dP < 0
        if dV < 0
            duty = duty_old + delta;
        else
            duty = duty_old - delta;
        end
    else
        if dV < 0
            duty = duty_old - delta;
        else
            duty = duty_old + delta;
        end
    end

    if Vbb < target 
        duty = (1e-3) + duty;
    elseif Vbb > target
        duty = (1e-3) - duty;
    else
        duty = duty_old;
    end

    % Limit duty cycle to min and max values
    duty = max(min(duty, duty_max), duty_min);

    % Update persistent variables
    duty_old = duty;
    Vpast = V;
    Ppast = P;
    Ipast = I;
    deltaw = delta;
end

== matlab function finalsimple_VER/Load profile/dynamic load test/Rover load/7 days ==
  data: u input; y output
function y = fcn(u)
    
    persistent a n
    if isempty(a)
        a = 0;
        n = 0;
    end
    
    % Update the output and the accumulated value
    y = u + a;
    a = y;
    
    % Increment the sample counter
    n = n + 1;
    
    % Reset the accumulation 
    if n >= 8400
        a = 0;
        n = 0;
    end
end

== matlab function finalsimple_VER/Load profile/dynamic load test/Rover load/next ==
  data: u input; y output
function y = fcn(u)
    
    persistent a sampleCount
    if isempty(a)
        a = 0;
        sampleCount = 0;
    end
    
    % Update the output and the accumulated value
    y = u + a;
    a = y;
    
    % Increment the sample counter
    sampleCount = sampleCount + 1;
    
    % Reset the accumulation after 24 samples
    if sampleCount >= 12
        a = 0;
        sampleCount = 0;
    end
end
